simulink model "funcionbonita"  (R2018a)
settings: Solver=VariableStepAuto  StartTime=0.0  StopTime=50  RelTol=1e-3
values from neighbouring files (symbols this model uses):
  A_0 = [0 -3.26931291643 0 0.71460251427 0 0 0 0 1 -0.0325743287495 0 -0.000548520916999 ... (64 elements, 8x8)]    [parametros.mat]    (also in twin_rotor_modelo_V1.m = eval(A_0))
  B_0 = [0 0 0 0 0 0 1190.47619048 0 0 0 0 0 ... (16 elements, 8x2)]    [parametros.mat]    (also in twin_rotor_modelo_V1.m = eval(B_0))
  C_0 = [1 0 0 0 0 1 0 0 0 0 0 0 ... (16 elements, 2x8)]    [parametros.mat]    (also in twin_rotor_modelo_V1.m = eval(C_0))
  u0 = [11.9668031953 -0.0853053139382]    [parametros.mat]    (also in twin_rotor_modelo_V1.m = [u_p_0;u_t_0])
  x0 = [0.0001 0 0 0 65.3284351132 -0.694344279837 0.788144659543 -0.00372302562915]    [parametros.mat]    (also in twin_rotor_modelo_V1.m = [phi_0; d_phi_0; theta_0; d_theta_0; w_p_0; w_t_0; i_p_0; i_)
settings Model: Creator=Gonzalo  LastModifiedBy=Gonzalo

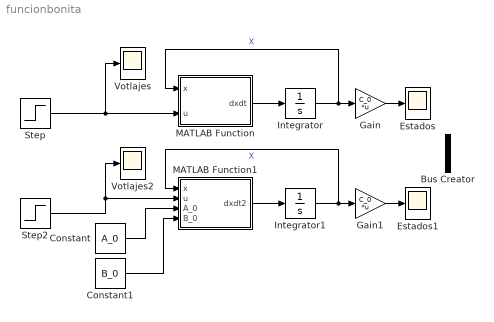
== system funcionbonita ==
  Bus Creator : BusCreator  Inputs=2
  Constant : Constant  Value=A_0
  Constant1 : Constant  Value=B_0
  Estados : Scope
  Estados1 : Scope
  Gain : Gain  Gain=C_0  Multiplication=Matrix(K*u)
  Gain1 : Gain  Gain=C_0  Multiplication=Matrix(K*u)
  Integrator : Integrator  InitialCondition=x0
  Integrator1 : Integrator  InitialCondition=x0
  MATLAB Function : MATLAB Function  TreatAsAtomicUnit=on
  MATLAB Function1 : MATLAB Function  TreatAsAtomicUnit=on
  Step : Step  Time=10  Before=u0  After=u0  SampleTime=0
  Step2 : Step  Time=10  Before=u0  After=u0  SampleTime=0
  Votlajes : Scope
  Votlajes2 : Scope
  wires:
  Step/1 -> MATLAB Function/2(u), Votlajes/1
  MATLAB Function/1(dxdt) -> Integrator/1
  Integrator/1 -> Gain/1, MATLAB Function/1(x)  "X"
  Gain/1 -> Estados/1
  Step2/1 -> MATLAB Function1/2(u), Votlajes2/1
  Integrator1/1 -> MATLAB Function1/1(x), Gain1/1  "X"
  Gain1/1 -> Estados1/1
  MATLAB Function1/1(dxdt2) -> Integrator1/1
  Constant/1 -> MATLAB Function1/3(A_0)
  Constant1/1 -> MATLAB Function1/4(B_0)

== matlab function funcionbonita/MATLAB Function1 ==
  data: x input; u input; dxdt2 output; A_0 input; B_0 input
function dxdt2 = funcion(x,u,A_0,B_0)
dxdt2 = A_0*x + B_0*u;

== matlab function funcionbonita/MATLAB Function ==
  data: x input; u input; dxdt output
function dxdt = func_f_x(x,u) 
phi = x(1);d_phi = x(2);theta = x(3);d_theta = x(4);w_p = x(5); w_t = x(6); i_p = x(7); i_t = x(8);
u_p = u(1); u_t = u(2);
dxdt = [d_phi;
(((2231553*cos(phi)^2)/4000000 + 6271303914229987/36028797018963968)*((3*d_phi)/250 - (27043227*cos(phi))/20000000 + (3022461*sin(phi))/2500000 + (1256252657407189*d_theta^2*sin(2*phi))/9007199254740992 + (2921964261275593*w_p*abs(w_p))/9223372036854775808))/((1566754414544131*cos(phi)*sin(phi))/9223372036854775808 - (1850992331451507*cos(phi)^2)/9007199254740992 + (3504602316272157*sin(phi)^2)/36893488147419103232 - 4621850957490069/72057594037927936) - (((1027*cos(phi))/25000 + (9189*sin(phi))/200000)*((6466506135038883*w_t*abs(w_t))/368934881474191032320 - (9*d_theta)/5000 + (9*d_phi^2*((9189*cos(phi))/200000 - (1027*sin(phi))/25000))/200 + (1507503188888627*d_phi*d_theta*sin(2*phi))/18014398509481984 + (7304910653188983*w_p*abs(w_p)*sin(phi))/368934881474191032320))/((1566754414544131*cos(phi)*sin(phi))/9223372036854775808 - (1850992331451507*cos(phi)^2)/9007199254740992 + (3504602316272157*sin(phi)^2)/36893488147419103232 - 4621850957490069/72057594037927936);
d_theta;
(((1027*cos(phi))/25000 + (9189*sin(phi))/200000)*((9*d_phi)/2500 - (81129681*cos(phi))/200000000 + (9067383*sin(phi))/25000000 + (1507503188888627*d_theta^2*sin(2*phi))/36028797018963968 + (438294639191339*w_p*abs(w_p))/4611686018427387904))/((1566754414544131*cos(phi)*sin(phi))/9223372036854775808 - (1850992331451507*cos(phi)^2)/9007199254740992 + (3504602316272157*sin(phi)^2)/36893488147419103232 - 4621850957490069/72057594037927936) - ((3177141253833869*w_t*abs(w_t))/73786976294838206464 - (4978621639436999*d_theta)/1125899906842624000 + (4978621639436999*d_phi^2*((9189*cos(phi))/200000 - (1027*sin(phi))/25000))/45035996273704960 + (7406705370233703*d_phi*d_theta*sin(2*phi))/36028797018963968 + (7178136850767151*w_p*abs(w_p)*sin(phi))/147573952589676412928)/((1566754414544131*cos(phi)*sin(phi))/9223372036854775808 - (1850992331451507*cos(phi)^2)/9007199254740992 + (3504602316272157*sin(phi)^2)/36893488147419103232 - 4621850957490069/72057594037927936);
(74600*i_p)/1083 - (300*w_p)/361;
(1492000*i_t)/10609 - (8000*w_t)/10609;
(25000*u_p)/21 - (75000*i_p)/7 - (1865*w_p)/21;
(25000*u_t)/21 - (75000*i_t)/7 - (1865*w_t)/21;
];
